simulink model "simulink_with_hdl"  (R2015a)
settings: Solver=ode45  StartTime=0.0  StopTime=1.0  RelTol=1e-3
libraries: dspsrcs4 x3
settings Model: Creator=vinicius.ls  LastModifiedBy=vinicius.ls
settings OptimizationCC: BlockReduction=off  ConditionallyExecuteInputs=off  InlineParams=on
settings DebuggingCC: AlgebraicLoopMsg=error
settings HardwareCC: ProdHWDeviceType=ASIC/FPGA->ASIC/FPGA  ProdEqTarget=off

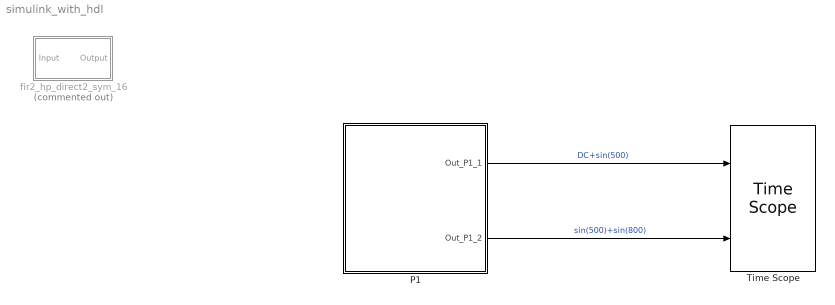
== system simulink_with_hdl ==
  P1 : Subsystem
  Time Scope : TimeScope  DefaultConfigurationName=spbscopes.TimeScopeBlockCfg  NumInputPorts=2
  fir2_hp_direct2_sym_16 : Subsystem  Tag=FilterWizardSubSystem  Commented=on
      settings: ErrorFcn=dspFilterRealizedInBasicElemsAlgLoopErrFcnCallback
  wires:
  P1/1(Out_P1_1) -> Time Scope/1  "DC+sin(500)"
  P1/2(Out_P1_2) -> Time Scope/2  "sin(500)+sin(800)"

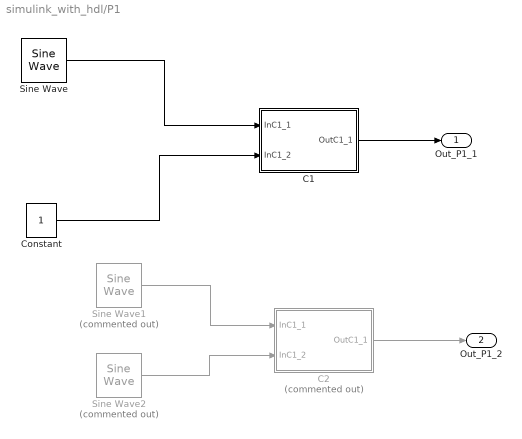
== system simulink_with_hdl/P1 ==
  C1 : Subsystem
  C2 : Subsystem  Commented=on
  Constant : Constant  VectorParams1D=off  OutDataTypeStr=Inherit: Inherit via back propagation
  Sine Wave : dspsrcs4/Sine Wave  Amplitude=1  Frequency=500  Phase=0  SampleMode=Discrete  OutComplex=Real  CompMethod=Table lookup  TableSize=Speed  SampleTime=1/8000  SamplesPerFrame=1  ResetState=Restart at time zero  dataType=Fixed-point  wordLen=16  udDataType=sfix(16)  fracBitsMode=Best precision  numFracBits=14  OutDataTypeStr=fixdt(1,16)  LastOutDataTypeStr=fixdt(1,16)
  Sine Wave1 : dspsrcs4/Sine Wave  Commented=on  Amplitude=1  Frequency=500  Phase=0  SampleMode=Discrete  OutComplex=Real  CompMethod=Trigonometric fcn  TableSize=Speed  SampleTime=1/8000  SamplesPerFrame=1  ResetState=Restart at time zero  dataType=double  wordLen=16  udDataType=sfix(16)  fracBitsMode=Best precision  numFracBits=15  OutDataTypeStr=double  LastOutDataTypeStr=double
  Sine Wave2 : dspsrcs4/Sine Wave  Commented=on  Amplitude=1  Frequency=800  Phase=0  SampleMode=Discrete  OutComplex=Real  CompMethod=Trigonometric fcn  TableSize=Speed  SampleTime=1/8000  SamplesPerFrame=1  ResetState=Restart at time zero  dataType=double  wordLen=16  udDataType=sfix(16)  fracBitsMode=Best precision  numFracBits=15  OutDataTypeStr=double  LastOutDataTypeStr=double
  Out_P1_1 : Outport
  Out_P1_2 : Outport  Port=2
  wires:
  Sine Wave/1 -> C1/1(InC1_1)
  Constant/1 -> C1/2(InC1_2)
  C1/1(OutC1_1) -> Out_P1_1/1
  Sine Wave1/1 -> C2/1(InC1_1)
  Sine Wave2/1 -> C2/2(InC1_2)
  C2/1(OutC1_1) -> Out_P1_2/1

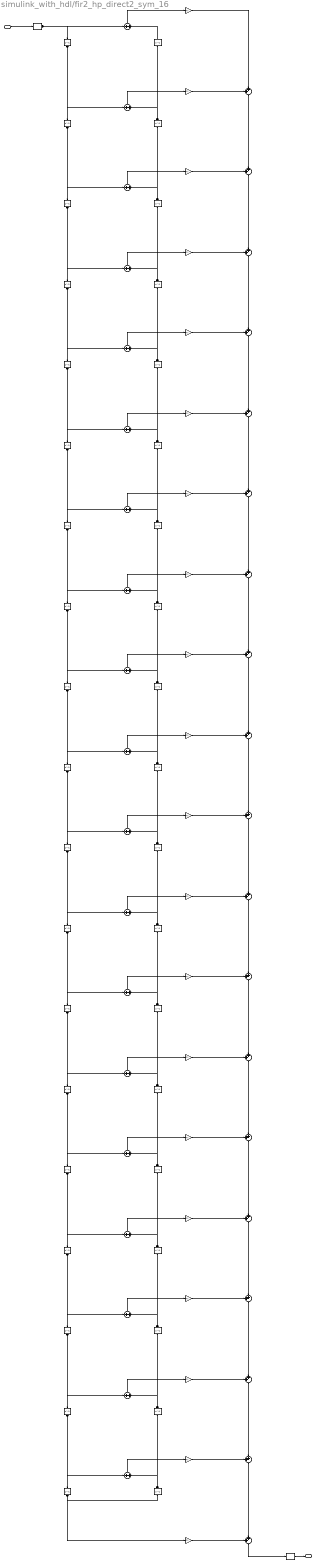
== system simulink_with_hdl/fir2_hp_direct2_sym_16 ==
  Input : Inport
  BodyDelayL{2..19} (18 alike) : Delay  DelayLength=1  InitialCondition=0  InputProcessing=Columns as channels (frame based)
  BodyDelayR{2..19} (18 alike) : Delay  DelayLength=1  InitialCondition=0  InputProcessing=Columns as channels (frame based)
  BodySumL{2..19} (18 alike) : Sum  Inputs=+|+  AccumDataTypeStr=fixdt(1,17,15)  OutDataTypeStr=fixdt(1,17,15)  RndMeth=Convergent
  BodySumR{2..19} (18 alike) : Sum  Inputs=++|  AccumDataTypeStr=fixdt(1,33,31)  OutDataTypeStr=fixdt(1,33,31)  RndMeth=Convergent
  ConvertIn : DataTypeConversion  OutDataTypeStr=fixdt(1,16,15)  RndMeth=Nearest  SaturateOnIntegerOverflow=on
  ConvertOut : DataTypeConversion  OutDataTypeStr=fixdt(1,33,31)  RndMeth=Convergent
  FootDelayL20 : Delay  DelayLength=1  InitialCondition=0  InputProcessing=Columns as channels (frame based)
  FootSumR20 : Sum  Inputs=++|  AccumDataTypeStr=fixdt(1,33,31)  OutDataTypeStr=fixdt(1,33,31)  RndMeth=Convergent
  HeadDelayR1 : Delay  DelayLength=1  InitialCondition=0  InputProcessing=Columns as channels (frame based)
  HeadSumL1 : Sum  Inputs=+|+  AccumDataTypeStr=fixdt(1,17,15)  OutDataTypeStr=fixdt(1,17,15)  RndMeth=Convergent
  h(1) : Gain  Gain=0.00619699398267406325  ParamDataTypeStr=fixdt(1,16,16)  OutDataTypeStr=fixdt(1,32,31)  RndMeth=Convergent
  h(10) : Gain  Gain=0.0030371422774610273  ParamDataTypeStr=fixdt(1,16,16)  OutDataTypeStr=fixdt(1,32,31)  RndMeth=Convergent
  h(11) : Gain  Gain=0.0266165572835444716  ParamDataTypeStr=fixdt(1,16,16)  OutDataTypeStr=fixdt(1,32,31)  RndMeth=Convergent
  h(12) : Gain  Gain=-0.0225179978188348277  ParamDataTypeStr=fixdt(1,16,16)  OutDataTypeStr=fixdt(1,32,31)  RndMeth=Convergent
  h(13) : Gain  Gain=-0.0206965844808010592  ParamDataTypeStr=fixdt(1,16,16)  OutDataTypeStr=fixdt(1,32,31)  RndMeth=Convergent
  h(14) : Gain  Gain=0.0464625395458445958  ParamDataTypeStr=fixdt(1,16,16)  OutDataTypeStr=fixdt(1,32,31)  RndMeth=Convergent
  h(15) : Gain  Gain=-0.00353161094216020719  ParamDataTypeStr=fixdt(1,16,16)  OutDataTypeStr=fixdt(1,32,31)  RndMeth=Convergent
  h(16) : Gain  Gain=-0.0697655318109630523  ParamDataTypeStr=fixdt(1,16,16)  OutDataTypeStr=fixdt(1,32,31)  RndMeth=Convergent
  h(17) : Gain  Gain=0.0621695057387276415  ParamDataTypeStr=fixdt(1,16,16)  OutDataTypeStr=fixdt(1,32,31)  RndMeth=Convergent
  h(18) : Gain  Gain=0.0867394766745781948  ParamDataTypeStr=fixdt(1,16,16)  OutDataTypeStr=fixdt(1,32,31)  RndMeth=Convergent
  h(19) : Gain  Gain=-0.293189641227315945  ParamDataTypeStr=fixdt(1,16,16)  OutDataTypeStr=fixdt(1,32,31)  RndMeth=Convergent
  h(2) : Gain  Gain=-0.00630024955810976842  ParamDataTypeStr=fixdt(1,16,16)  OutDataTypeStr=fixdt(1,32,31)  RndMeth=Convergent
  h(20) : Gain  Gain=0.390349619649230206  ParamDataTypeStr=fixdt(1,16,16)  OutDataTypeStr=fixdt(1,32,31)  RndMeth=Convergent
  h(3) : Gain  Gain=-0.00400200429052465466  ParamDataTypeStr=fixdt(1,16,16)  OutDataTypeStr=fixdt(1,32,31)  RndMeth=Convergent
  h(4) : Gain  Gain=0.0111238741446140366  ParamDataTypeStr=fixdt(1,16,16)  OutDataTypeStr=fixdt(1,32,31)  RndMeth=Convergent
  h(5) : Gain  Gain=-0.00230972163692039862  ParamDataTypeStr=fixdt(1,16,16)  OutDataTypeStr=fixdt(1,32,31)  RndMeth=Convergent
  h(6) : Gain  Gain=-0.0130229371939248467  ParamDataTypeStr=fixdt(1,16,16)  OutDataTypeStr=fixdt(1,32,31)  RndMeth=Convergent
  h(7) : Gain  Gain=0.0118778701746248931  ParamDataTypeStr=fixdt(1,16,16)  OutDataTypeStr=fixdt(1,32,31)  RndMeth=Convergent
  h(8) : Gain  Gain=0.00893550178570755825  ParamDataTypeStr=fixdt(1,16,16)  OutDataTypeStr=fixdt(1,32,31)  RndMeth=Convergent
  h(9) : Gain  Gain=-0.0216364126285692841  ParamDataTypeStr=fixdt(1,16,16)  OutDataTypeStr=fixdt(1,32,31)  RndMeth=Convergent
  Output : Outport
  wires:
  Input/1 -> ConvertIn/1
  HeadSumL1/1 -> h(1)/1
  h(1)/1 -> BodySumR2/2
  HeadDelayR1/1 -> HeadSumL1/2
  ConvertIn/1 -> HeadSumL1/1, BodyDelayL2/1
  BodyDelayL2/1 -> BodySumL2/1, BodyDelayL3/1
  BodySumL2/1 -> h(2)/1
  h(2)/1 -> BodySumR2/1
  BodyDelayR2/1 -> BodySumL2/2, HeadDelayR1/1
  BodySumR2/1 -> BodySumR3/2
  BodyDelayL3/1 -> BodySumL3/1, BodyDelayL4/1
  BodySumL3/1 -> h(3)/1
  h(3)/1 -> BodySumR3/1
  BodyDelayR3/1 -> BodySumL3/2, BodyDelayR2/1
  BodySumR3/1 -> BodySumR4/2
  BodyDelayL4/1 -> BodySumL4/1, BodyDelayL5/1
  BodySumL4/1 -> h(4)/1
  h(4)/1 -> BodySumR4/1
  BodyDelayR4/1 -> BodySumL4/2, BodyDelayR3/1
  BodySumR4/1 -> BodySumR5/2
  BodyDelayL5/1 -> BodySumL5/1, BodyDelayL6/1
  BodySumL5/1 -> h(5)/1
  h(5)/1 -> BodySumR5/1
  BodyDelayR5/1 -> BodySumL5/2, BodyDelayR4/1
  BodySumR5/1 -> BodySumR6/2
  BodyDelayL6/1 -> BodySumL6/1, BodyDelayL7/1
  BodySumL6/1 -> h(6)/1
  h(6)/1 -> BodySumR6/1
  BodyDelayR6/1 -> BodySumL6/2, BodyDelayR5/1
  BodySumR6/1 -> BodySumR7/2
  BodyDelayL7/1 -> BodySumL7/1, BodyDelayL8/1
  BodySumL7/1 -> h(7)/1
  h(7)/1 -> BodySumR7/1
  BodyDelayR7/1 -> BodySumL7/2, BodyDelayR6/1
  BodySumR7/1 -> BodySumR8/2
  BodyDelayL8/1 -> BodySumL8/1, BodyDelayL9/1
  BodySumL8/1 -> h(8)/1
  h(8)/1 -> BodySumR8/1
  BodyDelayR8/1 -> BodySumL8/2, BodyDelayR7/1
  BodySumR8/1 -> BodySumR9/2
  BodyDelayL9/1 -> BodySumL9/1, BodyDelayL10/1
  BodySumL9/1 -> h(9)/1
  h(9)/1 -> BodySumR9/1
  BodyDelayR9/1 -> BodySumL9/2, BodyDelayR8/1
  BodySumR9/1 -> BodySumR10/2
  BodyDelayL10/1 -> BodySumL10/1, BodyDelayL11/1
  BodySumL10/1 -> h(10)/1
  h(10)/1 -> BodySumR10/1
  BodyDelayR10/1 -> BodySumL10/2, BodyDelayR9/1
  BodySumR10/1 -> BodySumR11/2
  BodyDelayL11/1 -> BodySumL11/1, BodyDelayL12/1
  BodySumL11/1 -> h(11)/1
  h(11)/1 -> BodySumR11/1
  BodyDelayR11/1 -> BodySumL11/2, BodyDelayR10/1
  BodySumR11/1 -> BodySumR12/2
  BodyDelayL12/1 -> BodySumL12/1, BodyDelayL13/1
  BodySumL12/1 -> h(12)/1
  h(12)/1 -> BodySumR12/1
  BodyDelayR12/1 -> BodySumL12/2, BodyDelayR11/1
  BodySumR12/1 -> BodySumR13/2
  BodyDelayL13/1 -> BodySumL13/1, BodyDelayL14/1
  BodySumL13/1 -> h(13)/1
  h(13)/1 -> BodySumR13/1
  BodyDelayR13/1 -> BodySumL13/2, BodyDelayR12/1
  BodySumR13/1 -> BodySumR14/2
  BodyDelayL14/1 -> BodySumL14/1, BodyDelayL15/1
  BodySumL14/1 -> h(14)/1
  h(14)/1 -> BodySumR14/1
  BodyDelayR14/1 -> BodySumL14/2, BodyDelayR13/1
  BodySumR14/1 -> BodySumR15/2
  BodyDelayL15/1 -> BodySumL15/1, BodyDelayL16/1
  BodySumL15/1 -> h(15)/1
  h(15)/1 -> BodySumR15/1
  BodyDelayR15/1 -> BodySumL15/2, BodyDelayR14/1
  BodySumR15/1 -> BodySumR16/2
  BodyDelayL16/1 -> BodySumL16/1, BodyDelayL17/1
  BodySumL16/1 -> h(16)/1
  h(16)/1 -> BodySumR16/1
  BodyDelayR16/1 -> BodySumL16/2, BodyDelayR15/1
  BodySumR16/1 -> BodySumR17/2
  BodyDelayL17/1 -> BodySumL17/1, BodyDelayL18/1
  BodySumL17/1 -> h(17)/1
  h(17)/1 -> BodySumR17/1
  BodyDelayR17/1 -> BodySumL17/2, BodyDelayR16/1
  BodySumR17/1 -> BodySumR18/2
  BodyDelayL18/1 -> BodySumL18/1, BodyDelayL19/1
  BodySumL18/1 -> h(18)/1
  h(18)/1 -> BodySumR18/1
  BodyDelayR18/1 -> BodySumL18/2, BodyDelayR17/1
  BodySumR18/1 -> BodySumR19/2
  BodyDelayL19/1 -> BodySumL19/1, FootDelayL20/1
  BodySumL19/1 -> h(19)/1
  h(19)/1 -> BodySumR19/1
  BodyDelayR19/1 -> BodySumL19/2, BodyDelayR18/1
  BodySumR19/1 -> FootSumR20/2
  FootDelayL20/1 -> h(20)/1, BodyDelayR19/1
  h(20)/1 -> FootSumR20/1
  FootSumR20/1 -> ConvertOut/1
  ConvertOut/1 -> Output/1

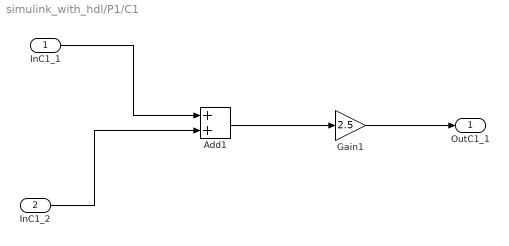
== system simulink_with_hdl/P1/C1 ==
  InC1_1 : Inport
  InC1_2 : Inport  Port=2
  Add1 : Sum
  Gain1 : Gain  Gain=2.5
  OutC1_1 : Outport
  wires:
  Add1/1 -> Gain1/1
  Gain1/1 -> OutC1_1/1
  InC1_2/1 -> Add1/2
  InC1_1/1 -> Add1/1

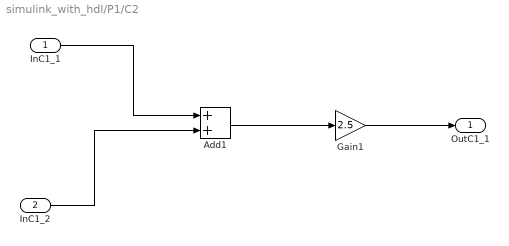
== system simulink_with_hdl/P1/C2 ==
  InC1_1 : Inport
  InC1_2 : Inport  Port=2
  Add1 : Sum
  Gain1 : Gain  Gain=2.5
  OutC1_1 : Outport
  wires:
  InC1_1/1 -> Add1/1
  InC1_2/1 -> Add1/2
  Gain1/1 -> OutC1_1/1
  Add1/1 -> Gain1/1
